simulink model "EST"  (R2022b)
settings: Solver=FixedStepAuto  StartTime=0.0  StopTime=stopt  FixedStep=deltat  MaxStep=0.05  RelTol=1e-3
InitFcn:
  | clear all;
  | close all;
  | clc;
  | 
  | % add the data and script directories
  | addpath('data','scripts');
  | 
  | % load the constants (units)
  | constants;
  | 
  | % load the simulation parameters
  | preprocessing;
StopFcn:
  | postprocessing;
values from neighbouring files (symbols this model uses):
  aExtraction = 0.1    [preprocessing.m]
  aInjection = 0.1    [preprocessing.m]
  bStorage = 1e-6/unit("s")    [preprocessing.m]
  EStorageInitial = 2.0*unit("kWh")    [preprocessing.m]
  EStorageMax = Eformula.*unit("kWh")    [preprocessing.m]
  EStorageMin = 0.0*unit("kWh")    [preprocessing.m]
settings Model: Creator=joche  LastModifiedBy=20234575
settings DataIOCC: SaveFormat=Array  SaveOutput=off  ReturnWorkspaceOutputs=off
settings ModelReferenceCC: EnableRefExpFcnMdlSchedulingChecks=on

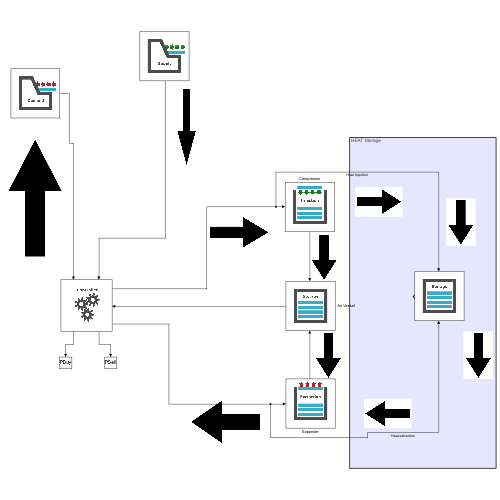
[thumbnail: Simulink's stored preview of the top-level diagram]
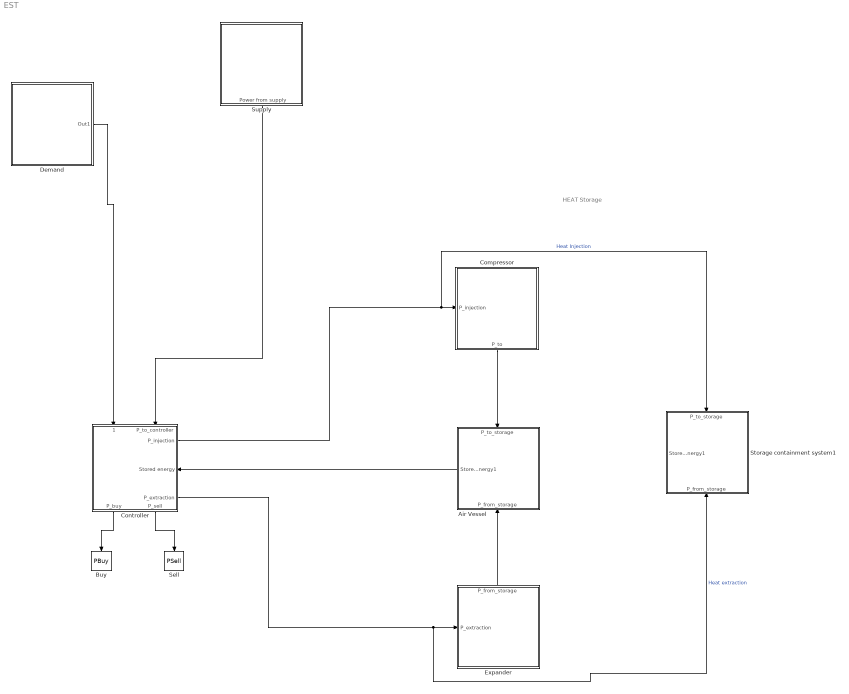
== system EST ==
  note: HEAT Storage
  Air Vessel : Subsystem
      settings: PortSchema="{\"entries\":[{\"content\":{\"sides\":[{\"content\":{\"connectorIds\":[\"Out1\"]},\"type\":\"ConnectorPlacement.EquallySpacedRectSide\",\"uuid\":\"0ba48424-33b9-4934-970f-64fe5d8b070e\"},{\"content\":{\"connectorIds\":[],\"side\":\"RIGHT\"},\"type\":\"ConnectorPlacement.EquallySpacedRectSide\",\"uuid\":\"9cde340f-8f39-4499-9a12-5e1623737660\"},{\"content\":{\"connectorIds\":[\"In1\"],\"side\":\"TOP\"},\"type\":\"ConnectorPlacement.EquallySpacedRectSide\",\"uuid\":\"2af8db04-7fd0-4902-8637-8dc00edb4598\"},{\"content\":{\"connectorIds\":[\"In2\"],\"side\":\"BOTTOM\"},\"type\":\"ConnectorPlacement.EquallySpacedRectSide\",\"uuid\":\"e21ea806-d777-41a3-a53f-556fae66854b\"}]},\"type\":\"ConnectorPlacement.EquallySpacedConnector\",\"uuid\":\"4e2ddb36-4db3-4ab4-858b-ebb8ccefeb1f\"}],\"packageUris\":[\"http://schema.mathworks.com/mf0/Connector/R2020b\"],\"version\":\"1.0\"}"
      mask Display: image('$imagefile'); % Use "Edit Image" on toolstrip to change.
  Buy : ToWorkspace  VariableName=PBuy  SampleTime=-1
  Compressor : Subsystem
      settings: PortSchema="{\"entries\":[{\"content\":{\"sides\":[{\"content\":{\"connectorIds\":[]},\"type\":\"ConnectorPlacement.EquallySpacedRectSide\",\"uuid\":\"05c5933d-55fc-4e06-853f-fc26d42905f9\"},{\"content\":{\"connectorIds\":[\"In1\"],\"side\":\"RIGHT\"},\"type\":\"ConnectorPlacement.EquallySpacedRectSide\",\"uuid\":\"327426c5-31d5-498b-a2bd-83e49353408c\"},{\"content\":{\"connectorIds\":[\"Out1\"],\"side\":\"TOP\"},\"type\":\"ConnectorPlacement.EquallySpacedRectSide\",\"uuid\":\"55306cf3-a3de-4385-a5ae-b8600ecdd5a2\"},{\"content\":{\"connectorIds\":[],\"side\":\"BOTTOM\"},\"type\":\"ConnectorPlacement.EquallySpacedRectSide\",\"uuid\":\"08fcc9c3-40d3-4ac6-b914-dfeef6039ffb\"}]},\"type\":\"ConnectorPlacement.EquallySpacedConnector\",\"uuid\":\"cb35d5ba-e8c6-462c-b7b2-fe8356d4b0a1\"}],\"packageUris\":[\"http://schema.mathworks.com/mf0/Connector/R2020b\"],\"version\":\"1.0\"}"
      mask Display: image('$imagefile'); % Use "Edit Image" on toolstrip to change.
  Controller : Subsystem
      settings: PortSchema="{\"entries\":[{\"content\":{\"sides\":[{\"content\":{\"connectorIds\":[]},\"type\":\"ConnectorPlacement.EquallySpacedRectSide\",\"uuid\":\"4daf33ce-c96a-4783-b5c4-228eed953e01\"},{\"content\":{\"connectorIds\":[\"Out1\",\"In3\",\"Out2\"],\"side\":\"RIGHT\"},\"type\":\"ConnectorPlacement.EquallySpacedRectSide\",\"uuid\":\"e9942e50-8467-4af8-b79b-80636cbc76e5\"},{\"content\":{\"connectorIds\":[\"In1\",\"In2\"],\"side\":\"TOP\"},\"type\":\"ConnectorPlacement.EquallySpacedRectSide\",\"uuid\":\"f315e931-d69b-4751-b712-f89c6c81baeb\"},{\"content\":{\"connectorIds\":[\"Out3\",\"Out4\"],\"side\":\"BOTTOM\"},\"type\":\"ConnectorPlacement.EquallySpacedRectSide\",\"uuid\":\"44715ee6-5cd5-4669-bcb9-5ed7c869bdb3\"}]},\"type\":\"ConnectorPlacement.EquallySpacedConnector\",\"uuid\":\"fff48899-944b-4064-b7d7-ecc12144fb48\"}],\"packageUris\":[\"http://schema.mathworks.com/mf0/Connector/R2020b\"],\"version\":\"1.0\"}"
      mask Display: image('$imagefile'); % Use "Edit Image" on toolstrip to change.
  Demand : Subsystem
      mask Display: image('$imagefile'); % Use "Edit Image" on toolstrip to change.
  Expander : Subsystem
      settings: PortSchema="{\"entries\":[{\"content\":{\"sides\":[{\"content\":{\"connectorIds\":[]},\"type\":\"ConnectorPlacement.EquallySpacedRectSide\",\"uuid\":\"05c5933d-55fc-4e06-853f-fc26d42905f9\"},{\"content\":{\"connectorIds\":[\"In1\"],\"side\":\"RIGHT\"},\"type\":\"ConnectorPlacement.EquallySpacedRectSide\",\"uuid\":\"327426c5-31d5-498b-a2bd-83e49353408c\"},{\"content\":{\"connectorIds\":[],\"side\":\"TOP\"},\"type\":\"ConnectorPlacement.EquallySpacedRectSide\",\"uuid\":\"55306cf3-a3de-4385-a5ae-b8600ecdd5a2\"},{\"content\":{\"connectorIds\":[\"Out1\"],\"side\":\"BOTTOM\"},\"type\":\"ConnectorPlacement.EquallySpacedRectSide\",\"uuid\":\"08fcc9c3-40d3-4ac6-b914-dfeef6039ffb\"}]},\"type\":\"ConnectorPlacement.EquallySpacedConnector\",\"uuid\":\"cb35d5ba-e8c6-462c-b7b2-fe8356d4b0a1\"}],\"packageUris\":[\"http://schema.mathworks.com/mf0/Connector/R2020b\"],\"version\":\"1.0\"}"
      mask Display: image('$imagefile'); % Use "Edit Image" on toolstrip to change.
  Sell : ToWorkspace  VariableName=PSell  SampleTime=-1
  Storage containment system1 : Subsystem
      settings: PortSchema="{\"entries\":[{\"content\":{\"sides\":[{\"content\":{\"connectorIds\":[\"Out1\"]},\"type\":\"ConnectorPlacement.EquallySpacedRectSide\",\"uuid\":\"0ba48424-33b9-4934-970f-64fe5d8b070e\"},{\"content\":{\"connectorIds\":[],\"side\":\"RIGHT\"},\"type\":\"ConnectorPlacement.EquallySpacedRectSide\",\"uuid\":\"9cde340f-8f39-4499-9a12-5e1623737660\"},{\"content\":{\"connectorIds\":[\"In1\"],\"side\":\"TOP\"},\"type\":\"ConnectorPlacement.EquallySpacedRectSide\",\"uuid\":\"2af8db04-7fd0-4902-8637-8dc00edb4598\"},{\"content\":{\"connectorIds\":[\"In2\"],\"side\":\"BOTTOM\"},\"type\":\"ConnectorPlacement.EquallySpacedRectSide\",\"uuid\":\"e21ea806-d777-41a3-a53f-556fae66854b\"}]},\"type\":\"ConnectorPlacement.EquallySpacedConnector\",\"uuid\":\"4e2ddb36-4db3-4ab4-858b-ebb8ccefeb1f\"}],\"packageUris\":[\"http://schema.mathworks.com/mf0/Connector/R2020b\"],\"version\":\"1.0\"}"
      mask Display: image('$imagefile'); % Use "Edit Image" on toolstrip to change.
  Supply : Subsystem
      settings: PortSchema="{\"entries\":[{\"content\":{\"sides\":[{\"content\":{\"connectorIds\":[]},\"type\":\"ConnectorPlacement.EquallySpacedRectSide\",\"uuid\":\"2887d8af-a352-4517-becd-f045dbeccadd\"},{\"content\":{\"connectorIds\":[],\"side\":\"RIGHT\"},\"type\":\"ConnectorPlacement.EquallySpacedRectSide\",\"uuid\":\"4593abfd-e950-4e99-9586-d3f76468ac22\"},{\"content\":{\"connectorIds\":[],\"side\":\"TOP\"},\"type\":\"ConnectorPlacement.EquallySpacedRectSide\",\"uuid\":\"9320404b-ee71-4176-be86-6fd94b9fdab6\"},{\"content\":{\"connectorIds\":[\"Out1\"],\"side\":\"BOTTOM\"},\"type\":\"ConnectorPlacement.EquallySpacedRectSide\",\"uuid\":\"d61fc422-b6dd-4076-b327-82d6d43f6fa4\"}]},\"type\":\"ConnectorPlacement.EquallySpacedConnector\",\"uuid\":\"abf755c7-92b4-4758-9a08-ed88957b2638\"}],\"packageUris\":[\"http://schema.mathworks.com/mf0/Connector/R2020b\"],\"version\":\"1.0\"}"
      mask Display: image('$imagefile'); % Use "Edit Image" on toolstrip to change.
  wires:
  Supply/1(Power from supply) -> Controller/2(P_to_controller)
  Demand/1(Out1) -> Controller/1(P_from_controller)
  Controller/4(P_sell) -> Sell/1
  Controller/2(P_extraction) -> Storage containment system1/2(P_from_storage), Expander/1(P_extraction)  "Heat extraction"
  Compressor/1(P_to) -> Air Vessel/1(P_to_storage)
  Expander/1(P_from_storage) -> Air Vessel/2(P_from_storage)
  Controller/1(P_injection) -> Storage containment system1/1(P_to_storage), Compressor/1(P_injection)  "Heat Injection"
  Controller/3(P_buy) -> Buy/1
  Air Vessel/1(Stored energy1) -> Controller/3(Stored energy)

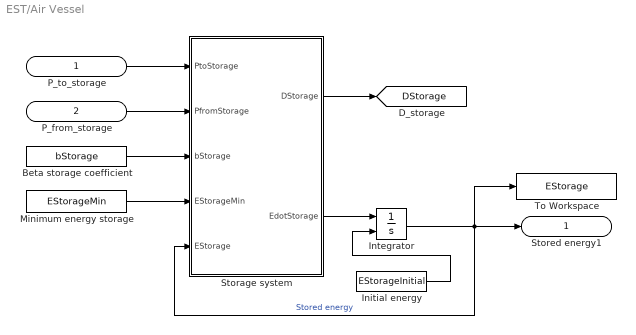
== system EST/Air Vessel ==
  P_to_storage : Inport
  P_from_storage : Inport  Port=2
  Beta storage coefficient : Constant  Value=bStorage
  Initial energy : Constant  Value=EStorageInitial
  Integrator : Integrator  InitialConditionSource=external
  Minimum energy storage : Constant  Value=EStorageMin
  Storage system : MATLAB Function  TreatAsAtomicUnit=on
  To Workspace : ToWorkspace  VariableName=EStorage  SampleTime=-1
  Stored energy1 : Outport
  tag scope: DStorage=global
  wires:
  P_from_storage/1 -> Storage system/2(PfromStorage)
  P_to_storage/1 -> Storage system/1(PtoStorage)
  Initial energy/1 -> Integrator/2
  Integrator/1 -> To Workspace/1, Storage system/5(EStorage), Stored energy1/1  "Stored energy"
  Storage system/1(DStorage) -> [DStorage]
  Beta storage coefficient/1 -> Storage system/3(bStorage)
  Storage system/2(EdotStorage) -> Integrator/1
  Minimum energy storage/1 -> Storage system/4(EStorageMin)

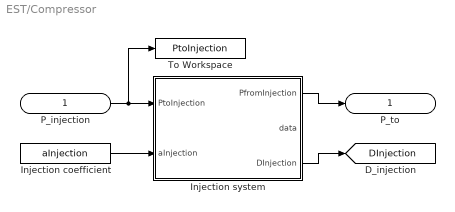
== system EST/Compressor ==
  P_injection : Inport
  Injection coefficient : Constant  Value=aInjection
  Injection system : MATLAB Function  TreatAsAtomicUnit=on
  To Workspace : ToWorkspace  VariableName=PtoInjection  SampleTime=-1
  P_to : Outport
  tag scope: DInjection=global
  wires:
  P_injection/1 -> To Workspace/1, Injection system/1(PtoInjection)
  Injection system/1(PfromInjection) -> P_to/1
  Injection coefficient/1 -> Injection system/2(aInjection)
  Injection system/3(DInjection) -> [DInjection]

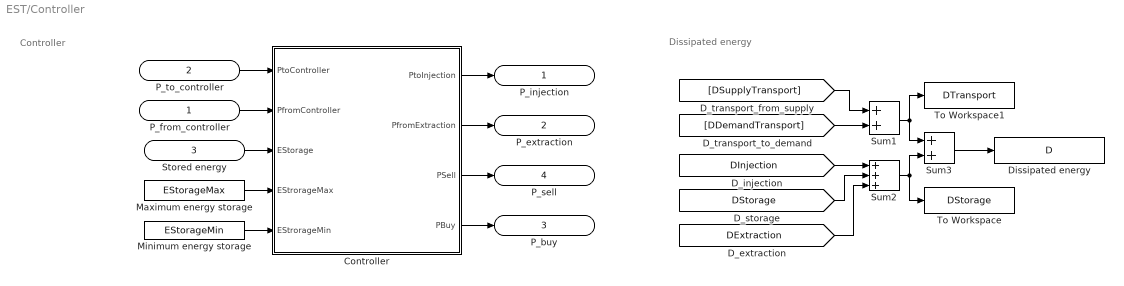
== system EST/Controller ==
  note: Dissipated energy
  note: Controller
  P_from_controller : Inport
  P_to_controller : Inport  Port=2
  Stored energy : Inport  Port=3
  Controller : MATLAB Function  TreatAsAtomicUnit=on
  Dissipated energy : ToWorkspace  VariableName=D  SampleTime=-1
  Maximum energy storage : Constant  Value=EStorageMax
  Minimum energy storage : Constant  Value=EStorageMin
  Sum1 : Sum
  Sum2 : Sum  Inputs=+++
  Sum3 : Sum
  To Workspace : ToWorkspace  VariableName=DStorage  SampleTime=-1
  To Workspace1 : ToWorkspace  VariableName=DTransport  SampleTime=-1
  P_injection : Outport
  P_extraction : Outport  Port=2
  P_buy : Outport  Port=3
  P_sell : Outport  Port=4
  wires:
  P_from_controller/1 -> Controller/2(PfromController)
  Controller/2(PfromExtraction) -> P_extraction/1
  Controller/3(PSell) -> P_sell/1
  Controller/4(PBuy) -> P_buy/1
  Minimum energy storage/1 -> Controller/5(EStrorageMin)
  Maximum energy storage/1 -> Controller/4(EStrorageMax)
  P_to_controller/1 -> Controller/1(PtoController)
  Controller/1(PtoInjection) -> P_injection/1
  Stored energy/1 -> Controller/3(EStorage)
  [DDemandTransport] -> Sum1/2
  [DSupplyTransport] -> Sum1/1
  [DInjection] -> Sum2/1
  [DStorage] -> Sum2/2
  [DExtraction] -> Sum2/3
  Sum2/1 -> To Workspace/1, Sum3/2
  Sum1/1 -> To Workspace1/1, Sum3/1
  Sum3/1 -> Dissipated energy/1

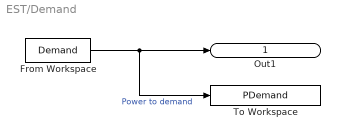
== system EST/Demand ==
  From Workspace : FromWorkspace  VariableName=Demand  OutputAfterFinalValue=Setting to zero
  To Workspace : ToWorkspace  VariableName=PDemand  SampleTime=-1
  Out1 : Outport
  wires:
  From Workspace/1 -> To Workspace/1, Out1/1  "Power to demand"

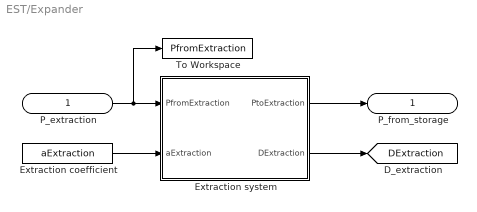
== system EST/Expander ==
  P_extraction : Inport
  Extraction coefficient : Constant  Value=aExtraction
  Extraction system : MATLAB Function  TreatAsAtomicUnit=on
  To Workspace : ToWorkspace  VariableName=PfromExtraction  SampleTime=-1
  P_from_storage : Outport
  tag scope: DExtraction=global
  wires:
  P_extraction/1 -> To Workspace/1, Extraction system/1(PfromExtraction)
  Extraction system/1(PtoExtraction) -> P_from_storage/1
  Extraction coefficient/1 -> Extraction system/2(aExtraction)
  Extraction system/2(DExtraction) -> [DExtraction]

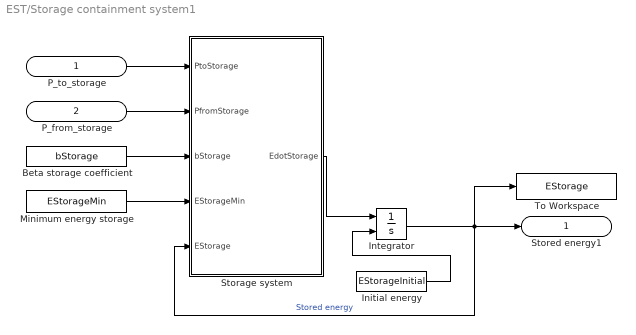
== system EST/Storage containment system1 ==
  P_to_storage : Inport
  P_from_storage : Inport  Port=2
  Beta storage coefficient : Constant  Value=bStorage
  Initial energy : Constant  Value=EStorageInitial
  Integrator : Integrator  InitialConditionSource=external
  Minimum energy storage : Constant  Value=EStorageMin
  Storage system : MATLAB Function  TreatAsAtomicUnit=on
  To Workspace : ToWorkspace  VariableName=EStorage  SampleTime=-1
  Stored energy1 : Outport
  wires:
  P_from_storage/1 -> Storage system/2(PfromStorage)
  P_to_storage/1 -> Storage system/1(PtoStorage)
  Initial energy/1 -> Integrator/2
  Integrator/1 -> To Workspace/1, Storage system/5(EStorage), Stored energy1/1  "Stored energy"
  Beta storage coefficient/1 -> Storage system/3(bStorage)
  Storage system/1(EdotStorage) -> Integrator/1
  Minimum energy storage/1 -> Storage system/4(EStorageMin)

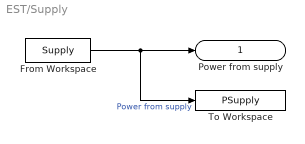
== system EST/Supply ==
  From Workspace : FromWorkspace  VariableName=Supply  OutputAfterFinalValue=Setting to zero
  To Workspace : ToWorkspace  VariableName=PSupply  SampleTime=-1
  Power from supply : Outport
  wires:
  From Workspace/1 -> To Workspace/1, Power from supply/1  "Power from supply"

== matlab function EST/Compressor/Injection system ==
  data: PtoInjection input; PfromInjection output; data output; aInjection input; DInjection output
function [PfromInjection, data, DInjection] = injection(PtoInjection, aInjection)
    DInjection = aInjection * PtoInjection;
    PfromInjection = PtoInjection - DInjection;

== matlab function EST/Storage containment system1/Storage system ==
  data: EdotStorage output; PtoStorage input; PfromStorage input; bStorage input; EStorageMin input; EStorage input
function EdotStorage = Storage(PtoStorage, PfromStorage, bStorage, EStorageMin, EStorage)
    DStorage = bStorage * (EStorage-EStorageMin);
    EdotStorage = PtoStorage - PfromStorage - DStorage;

== matlab function EST/Controller/Controller ==
  data: PtoInjection output; PfromExtraction output; PSell output; PBuy output; PtoController input; PfromController input; EStorage input; EStrorageMax input; EStrorageMin input
function [PtoInjection, PfromExtraction, PSell, PBuy] = controller(PtoController, PfromController, EStorage, EStrorageMax, EStrorageMin)
    
    %% Power surplus or deficit

    deltaP = PtoController - PfromController;

    % Power surplus
    if deltaP >= 0

        %% Storage injection

        % Storage system is not full
        if EStorage < EStrorageMax 

            PtoInjection = deltaP;

        % Storage system is full
        else
            PtoInjection = 0;
        end

        %% Storage extraction

        PfromExtraction = 0;

        %% Load-balancing
        PSell   = deltaP - PtoInjection;
        PBuy    = 0;

    % Power deficit
    else

        %% Storage injection

        PtoInjection = 0;

        %% Storage extraction

        % Storage system is not empty
        if EStorage > EStrorageMin

            PfromExtraction = -deltaP;

        % Storage system is empty
        else
            PfromExtraction = 0;
        end

        %% Load-balancing

        PSell = 0;
        PBuy  = -deltaP - PfromExtraction;
    end

== matlab function EST/Expander/Extraction system ==
  data: PfromExtraction input; PtoExtraction output; aExtraction input; DExtraction output
function [PtoExtraction, DExtraction] = extraction(PfromExtraction, aExtraction)
    DExtraction = aExtraction / (1-aExtraction) * PfromExtraction;
    PtoExtraction = PfromExtraction + DExtraction;

== matlab function EST/Air Vessel/Storage system ==
  data: DStorage output; EdotStorage output; PtoStorage input; PfromStorage input; bStorage input; EStorageMin input; EStorage input
function [DStorage, EdotStorage]= Storage(PtoStorage, PfromStorage, bStorage, EStorageMin, EStorage)
    DStorage = bStorage * (EStorage-EStorageMin);
    EdotStorage = PtoStorage - PfromStorage - DStorage;
